simulink model "prediction_slx"  (R2024a)
settings: Solver=VariableStepAuto  StartTime=0.0  StopTime=10.0  RelTol=1e-3
undefined symbols (not defined in the file or in its folder): torque_input1_sm
settings Model: Creator=amazon  LastModifiedBy=amazon

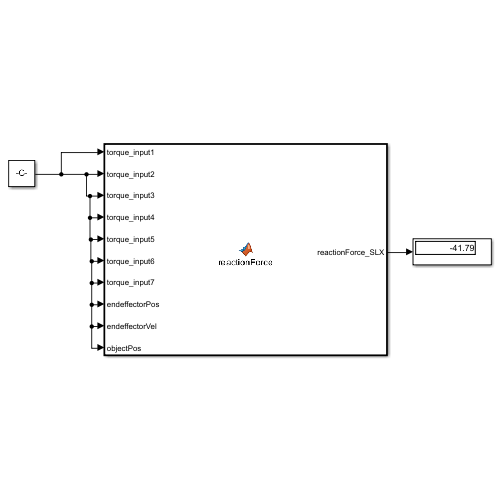
[thumbnail: Simulink's stored preview of the top-level diagram]
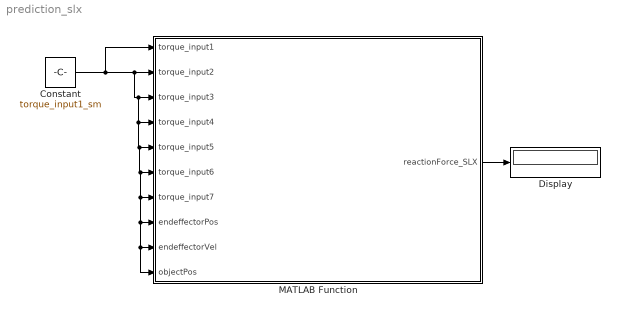
== system prediction_slx ==
  Constant : Constant  Value=torque_input1_sm
  Display : Display
  MATLAB Function : MATLAB Function  TreatAsAtomicUnit=on
  wires:
  MATLAB Function/1(reactionForce_SLX) -> Display/1
  Constant/1 -> MATLAB Function/1(torque_input1), MATLAB Function/10(objectPos), MATLAB Function/9(endeffectorVel), MATLAB Function/8(endeffectorPos), MATLAB Function/7(torque_input7), MATLAB Function/6(torque_input6), MATLAB Function/5(torque_input5), MATLAB Function/4(torque_input4), MATLAB Function/3(torque_input3), MATLAB Function/2(torque_input2)

== matlab function prediction_slx/MATLAB Function ==
  data: torque_input1 input; reactionForce_SLX output; torque_input2 input; torque_input3 input; torque_input4 input; torque_input5 input; torque_input6 input; torque_input7 input; endeffectorPos input; endeffectorVel input; objectPos input
function reactionForce_SLX  = reactionForce(torque_input1, torque_input2, torque_input3, torque_input4, torque_input5, torque_input6, torque_input7, endeffectorPos, endeffectorVel, objectPos)
    coder.extrinsic('predict_reactionForce');
    reactionForce_SLX = 0
    % Create the input array
    new_data = [torque_input1, torque_input2, torque_input3, torque_input4, torque_input5, torque_input6, torque_input7, endeffectorPos, endeffectorVel, objectPos];
    
    % Call the predict_rgb function
    reactionForce_SLX = predict_reactionForce(new_data);
end
